simulink model "tres_threeservos"  (Simulink 8.3)
settings: Solver=ode45  StartTime=0.0  StopTime=0.06  RelTol=1e-3
InitFcn:
  | clear functions
libraries: tres_simulink_blockset x4
settings Model: Creator=anton  LastModifiedBy=matteo  ExtModeTrigMode=oneshot  ExtModeArmWhenConnect=off  ExtModeAutoUpdateStatusClock=off
settings DataIOCC: LimitDataPoints=off
settings OptimizationCC: BlockReduction=off  BooleanDataType=off  InlineParams=on  ExpressionDepthLimit=2147483647
settings DebuggingCC: SaveWithParameterizedLinksMsg=none  SignalResolutionControl=TryResolveAllWithWarning  SolverPrmCheckMsg=none  MultiTaskDSMMsg=warning  MultiTaskCondExecSysMsg=none  FcnCallInpInsideContextMsg=UseLocalSettings  StrictBusMsg=None
settings HardwareCC: TargetUnknown=on
settings RTWCC: IncludeERTFirstTime=on

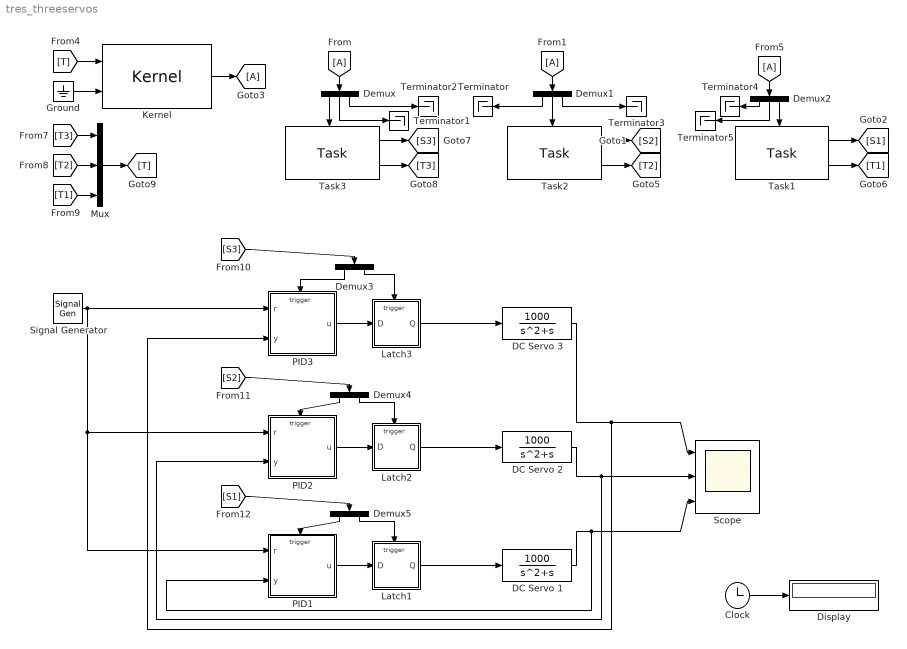
== system tres_threeservos ==
  Clock : Clock
  DC Servo 1 : TransferFcn  Numerator=[1000]  Denominator=[1 1 0]
  DC Servo 2 : TransferFcn  Numerator=[1000]  Denominator=[1 1 0]
  DC Servo 3 : TransferFcn  Numerator=[1000]  Denominator=[1 1 0]
  Demux : Demux  Outputs=3
  Demux1 : Demux  Outputs=3
  Demux2 : Demux  Outputs=3
  Demux3 : Demux  Outputs=2
  Demux4 : Demux  Outputs=2
  Demux5 : Demux  Outputs=2
  Display : Display
  Ground : Ground
  Kernel : tres_simulink_blockset/Kernel  taskset_descr_name=task_set_descr  scheduling_policy=DEADLINE_MONOTONIC  dead_miss_rule=Continue  time_res=Milli_Seconds  core_num=1  under_engine=RTSIM
  Latch1 : Subsystem  TreatAsAtomicUnit=on
  Latch2 : Subsystem  TreatAsAtomicUnit=on
  Latch3 : Subsystem  TreatAsAtomicUnit=on
  Mux : Mux  Inputs=3
  PID1 : Subsystem  TreatAsAtomicUnit=on
  PID2 : Subsystem  TreatAsAtomicUnit=on
  PID3 : Subsystem  TreatAsAtomicUnit=on
  Scope : Scope  NumInputPorts=3
      settings: YMin=-5~-5~-5  YMax=5~5~5
  Signal Generator : SignalGenerator  WaveForm=square  Frequency=1.5
  Task1 : tres_simulink_blockset/Task  conf_name=t1_descr
  Task2 : tres_simulink_blockset/Task  conf_name=t2_descr
  Task3 : tres_simulink_blockset/Task  conf_name=t3_descr
  Terminator{,1..5} (6 alike) : Terminator
  wires:
  Clock/1 -> Display/1
  Signal Generator/1 -> PID3/1(r), PID1/1(r), PID2/1(r)
  DC Servo 3/1 -> PID3/2(y), Scope/1
  DC Servo 2/1 -> PID2/2(y), Scope/2
  DC Servo 1/1 -> PID1/2(y), Scope/3
  PID3/1(u) -> Latch3/1(D)
  Latch3/1(Q) -> DC Servo 3/1
  PID2/1(u) -> Latch2/1(D)
  Latch2/1(Q) -> DC Servo 2/1
  PID1/1(u) -> Latch1/1(D)
  Latch1/1(Q) -> DC Servo 1/1
  [T] -> Kernel/1
  Kernel/1 -> [A]
  [A] -> Demux/1
  Demux/1 -> Task3/Trigger
  Demux/2 -> Terminator1/1
  Task3/2 -> [T3]
  Task3/1 -> [S3]
  Demux/3 -> Terminator2/1
  [A] -> Demux1/1
  Demux1/2 -> Task2/Trigger
  Demux1/1 -> Terminator/1
  Task2/2 -> [T2]
  Task2/1 -> [S2]
  Demux1/3 -> Terminator3/1
  [A] -> Demux2/1
  Demux2/1 -> Terminator4/1
  Task1/2 -> [T1]
  Task1/1 -> [S1]
  Demux2/2 -> Terminator5/1
  Demux2/3 -> Task1/Trigger
  [T3] -> Mux/1
  [T2] -> Mux/2
  Mux/1 -> [T]
  [T1] -> Mux/3
  [S3] -> Demux3/1
  Demux3/1 -> PID3/Trigger
  Demux3/2 -> Latch3/Trigger
  [S2] -> Demux4/1
  Demux4/1 -> PID2/Trigger
  Demux4/2 -> Latch2/Trigger
  Demux5/1 -> PID1/Trigger
  Demux5/2 -> Latch1/Trigger
  [S1] -> Demux5/1
  Ground/1 -> Kernel/2

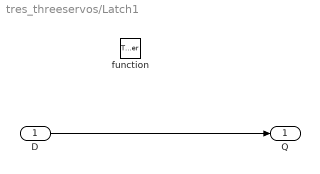
== system tres_threeservos/Latch1 ==
  D : Inport
  function : TriggerPort  TriggerType=function-call
  Q : Outport
  wires:
  D/1 -> Q/1

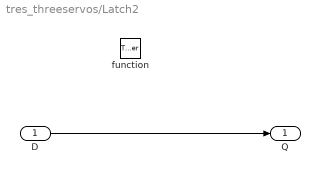
== system tres_threeservos/Latch2 ==
  D : Inport
  function : TriggerPort  TriggerType=function-call
  Q : Outport
  wires:
  D/1 -> Q/1

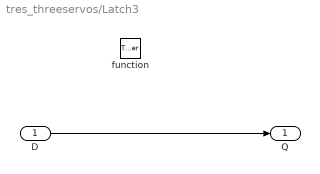
== system tres_threeservos/Latch3 ==
  D : Inport
  function : TriggerPort  TriggerType=function-call
  Q : Outport
  wires:
  D/1 -> Q/1

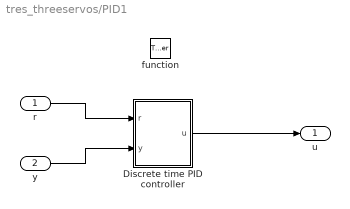
== system tres_threeservos/PID1 ==
  r : Inport
  y : Inport  Port=2
  function : TriggerPort  TriggerType=function-call
  Discrete time PID controller : Subsystem  mask{K=0.96, Ti=0.12, Td=0.049, beta=0.5, N=10, h=0.006}
  u : Outport
  wires:
  r/1 -> Discrete time PID controller/1(r)
  Discrete time PID controller/1(u) -> u/1
  y/1 -> Discrete time PID controller/2(y)

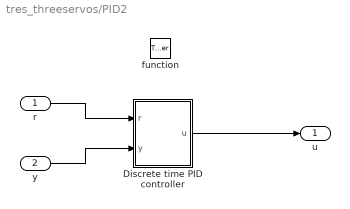
== system tres_threeservos/PID2 ==
  r : Inport
  y : Inport  Port=2
  function : TriggerPort  TriggerType=function-call
  Discrete time PID controller : Subsystem  mask{K=0.96, Ti=0.12, Td=0.049, beta=0.5, N=10, h=0.005}
  u : Outport
  wires:
  r/1 -> Discrete time PID controller/1(r)
  Discrete time PID controller/1(u) -> u/1
  y/1 -> Discrete time PID controller/2(y)

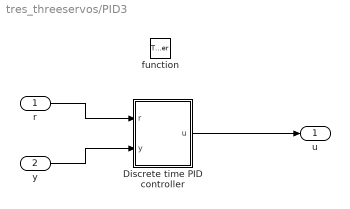
== system tres_threeservos/PID3 ==
  r : Inport
  y : Inport  Port=2
  function : TriggerPort  TriggerType=function-call
  Discrete time PID controller : Subsystem  mask{K=0.96, Ti=0.12, Td=0.049, beta=0.5, N=10, h=0.004}
  u : Outport
  wires:
  r/1 -> Discrete time PID controller/1(r)
  Discrete time PID controller/1(u) -> u/1
  y/1 -> Discrete time PID controller/2(y)

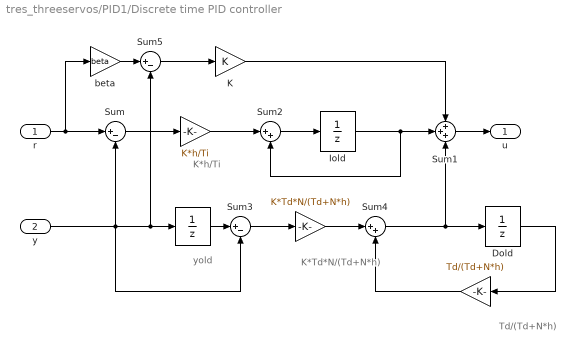
== system tres_threeservos/PID1/Discrete time PID controller ==
  note: K*h/Ti
  note: K*Td*N/(Td+N*h)
  note: Td/(Td+N*h)
  note: yold
  r : Inport
  y : Inport  Port=2
  " " : UnitDelay  SampleTime=-1
  "   " : Gain  Gain=K*h/Ti  SaturateOnIntegerOverflow=on  OutDataTypeStr=Inherit: Same as input  ParamDataTypeStr=Inherit: Same as input
  "             " : Gain  Gain=K*Td*N/(Td+N*h)  SaturateOnIntegerOverflow=on  OutDataTypeStr=Inherit: Same as input  ParamDataTypeStr=Inherit: Same as input
  "              " : Gain  Gain=Td/(Td+N*h)  SaturateOnIntegerOverflow=on  OutDataTypeStr=Inherit: Same as input  ParamDataTypeStr=Inherit: Same as input
  Dold : UnitDelay  SampleTime=-1
  "Iold " : UnitDelay  SampleTime=-1
  K : Gain  Gain=K  SaturateOnIntegerOverflow=on  OutDataTypeStr=Inherit: Same as input  ParamDataTypeStr=Inherit: Same as input
  Sum : Sum  Inputs=|+-  SaturateOnIntegerOverflow=on  InputSameDT=on  OutDataTypeStr=Inherit: Same as first input
  Sum1 : Sum  Inputs=+++  SaturateOnIntegerOverflow=on  InputSameDT=on  OutDataTypeStr=Inherit: Same as first input
  Sum2 : Sum  Inputs=|++  SaturateOnIntegerOverflow=on  InputSameDT=on  OutDataTypeStr=Inherit: Same as first input
  Sum3 : Sum  Inputs=|+-  SaturateOnIntegerOverflow=on  InputSameDT=on  OutDataTypeStr=Inherit: Same as first input
  Sum4 : Sum  Inputs=|++  SaturateOnIntegerOverflow=on  InputSameDT=on  OutDataTypeStr=Inherit: Same as first input
  Sum5 : Sum  Inputs=|+-  SaturateOnIntegerOverflow=on  InputSameDT=on  OutDataTypeStr=Inherit: Same as first input
  beta : Gain  Gain=beta  SaturateOnIntegerOverflow=on  OutDataTypeStr=Inherit: Same as input  ParamDataTypeStr=Inherit: Same as input
  u : Outport
  wires:
  y/1 -> Sum/2, Sum3/2, " "/1, Sum5/2
  r/1 -> Sum/1, beta/1
  Sum1/1 -> u/1
  K/1 -> Sum1/1
  Sum2/1 -> "Iold "/1
  Dold/1 -> "              "/1
  "             "/1 -> Sum4/1
  Sum3/1 -> "             "/1
  Sum4/1 -> Dold/1, Sum1/3
  " "/1 -> Sum3/1
  "Iold "/1 -> Sum2/2, Sum1/2
  "   "/1 -> Sum2/1
  Sum/1 -> "   "/1
  "              "/1 -> Sum4/2
  beta/1 -> Sum5/1
  Sum5/1 -> K/1

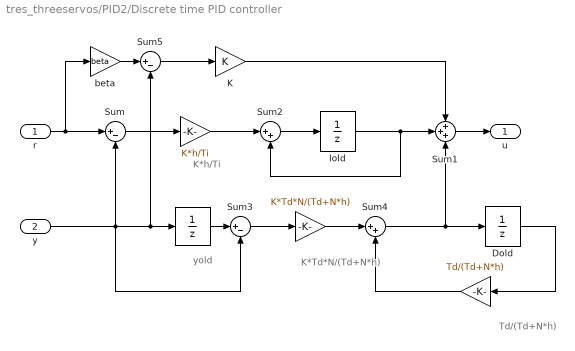
== system tres_threeservos/PID2/Discrete time PID controller ==
  note: K*h/Ti
  note: K*Td*N/(Td+N*h)
  note: Td/(Td+N*h)
  note: yold
  r : Inport
  y : Inport  Port=2
  " " : UnitDelay  SampleTime=-1
  "   " : Gain  Gain=K*h/Ti  SaturateOnIntegerOverflow=on  OutDataTypeStr=Inherit: Same as input  ParamDataTypeStr=Inherit: Same as input
  "             " : Gain  Gain=K*Td*N/(Td+N*h)  SaturateOnIntegerOverflow=on  OutDataTypeStr=Inherit: Same as input  ParamDataTypeStr=Inherit: Same as input
  "              " : Gain  Gain=Td/(Td+N*h)  SaturateOnIntegerOverflow=on  OutDataTypeStr=Inherit: Same as input  ParamDataTypeStr=Inherit: Same as input
  Dold : UnitDelay  SampleTime=-1
  "Iold " : UnitDelay  SampleTime=-1
  K : Gain  Gain=K  SaturateOnIntegerOverflow=on  OutDataTypeStr=Inherit: Same as input  ParamDataTypeStr=Inherit: Same as input
  Sum : Sum  Inputs=|+-  SaturateOnIntegerOverflow=on  InputSameDT=on  OutDataTypeStr=Inherit: Same as first input
  Sum1 : Sum  Inputs=+++  SaturateOnIntegerOverflow=on  InputSameDT=on  OutDataTypeStr=Inherit: Same as first input
  Sum2 : Sum  Inputs=|++  SaturateOnIntegerOverflow=on  InputSameDT=on  OutDataTypeStr=Inherit: Same as first input
  Sum3 : Sum  Inputs=|+-  SaturateOnIntegerOverflow=on  InputSameDT=on  OutDataTypeStr=Inherit: Same as first input
  Sum4 : Sum  Inputs=|++  SaturateOnIntegerOverflow=on  InputSameDT=on  OutDataTypeStr=Inherit: Same as first input
  Sum5 : Sum  Inputs=|+-  SaturateOnIntegerOverflow=on  InputSameDT=on  OutDataTypeStr=Inherit: Same as first input
  beta : Gain  Gain=beta  SaturateOnIntegerOverflow=on  OutDataTypeStr=Inherit: Same as input  ParamDataTypeStr=Inherit: Same as input
  u : Outport
  wires:
  y/1 -> Sum/2, Sum3/2, " "/1, Sum5/2
  r/1 -> Sum/1, beta/1
  Sum1/1 -> u/1
  K/1 -> Sum1/1
  Sum2/1 -> "Iold "/1
  Dold/1 -> "              "/1
  "             "/1 -> Sum4/1
  Sum3/1 -> "             "/1
  Sum4/1 -> Dold/1, Sum1/3
  " "/1 -> Sum3/1
  "Iold "/1 -> Sum2/2, Sum1/2
  "   "/1 -> Sum2/1
  Sum/1 -> "   "/1
  "              "/1 -> Sum4/2
  beta/1 -> Sum5/1
  Sum5/1 -> K/1

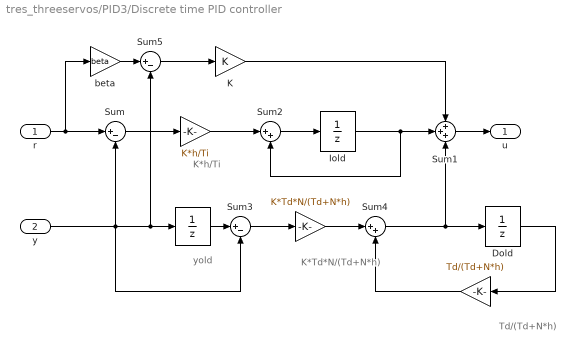
== system tres_threeservos/PID3/Discrete time PID controller ==
  note: K*h/Ti
  note: K*Td*N/(Td+N*h)
  note: Td/(Td+N*h)
  note: yold
  r : Inport
  y : Inport  Port=2
  " " : UnitDelay  SampleTime=-1
  "   " : Gain  Gain=K*h/Ti  SaturateOnIntegerOverflow=on  OutDataTypeStr=Inherit: Same as input  ParamDataTypeStr=Inherit: Same as input
  "             " : Gain  Gain=K*Td*N/(Td+N*h)  SaturateOnIntegerOverflow=on  OutDataTypeStr=Inherit: Same as input  ParamDataTypeStr=Inherit: Same as input
  "              " : Gain  Gain=Td/(Td+N*h)  SaturateOnIntegerOverflow=on  OutDataTypeStr=Inherit: Same as input  ParamDataTypeStr=Inherit: Same as input
  Dold : UnitDelay  SampleTime=-1
  "Iold " : UnitDelay  SampleTime=-1
  K : Gain  Gain=K  SaturateOnIntegerOverflow=on  OutDataTypeStr=Inherit: Same as input  ParamDataTypeStr=Inherit: Same as input
  Sum : Sum  Inputs=|+-  SaturateOnIntegerOverflow=on  InputSameDT=on  OutDataTypeStr=Inherit: Same as first input
  Sum1 : Sum  Inputs=+++  SaturateOnIntegerOverflow=on  InputSameDT=on  OutDataTypeStr=Inherit: Same as first input
  Sum2 : Sum  Inputs=|++  SaturateOnIntegerOverflow=on  InputSameDT=on  OutDataTypeStr=Inherit: Same as first input
  Sum3 : Sum  Inputs=|+-  SaturateOnIntegerOverflow=on  InputSameDT=on  OutDataTypeStr=Inherit: Same as first input
  Sum4 : Sum  Inputs=|++  SaturateOnIntegerOverflow=on  InputSameDT=on  OutDataTypeStr=Inherit: Same as first input
  Sum5 : Sum  Inputs=|+-  SaturateOnIntegerOverflow=on  InputSameDT=on  OutDataTypeStr=Inherit: Same as first input
  beta : Gain  Gain=beta  SaturateOnIntegerOverflow=on  OutDataTypeStr=Inherit: Same as input  ParamDataTypeStr=Inherit: Same as input
  u : Outport
  wires:
  y/1 -> Sum/2, Sum3/2, " "/1, Sum5/2
  r/1 -> Sum/1, beta/1
  Sum1/1 -> u/1
  K/1 -> Sum1/1
  Sum2/1 -> "Iold "/1
  Dold/1 -> "              "/1
  "             "/1 -> Sum4/1
  Sum3/1 -> "             "/1
  Sum4/1 -> Dold/1, Sum1/3
  " "/1 -> Sum3/1
  "Iold "/1 -> Sum2/2, Sum1/2
  "   "/1 -> Sum2/1
  Sum/1 -> "   "/1
  "              "/1 -> Sum4/2
  beta/1 -> Sum5/1
  Sum5/1 -> K/1
